simulink model "videomodel_V1"  (R2021a)
settings: Solver=VariableStepAuto  StartTime=0.0  StopTime=10.0  RelTol=1e-3
libraries: vexarmcortexlib x19, vexcommonlib x4
settings Model: Creator=Mihai Nicoara  LastModifiedBy=Mihai Nicoara

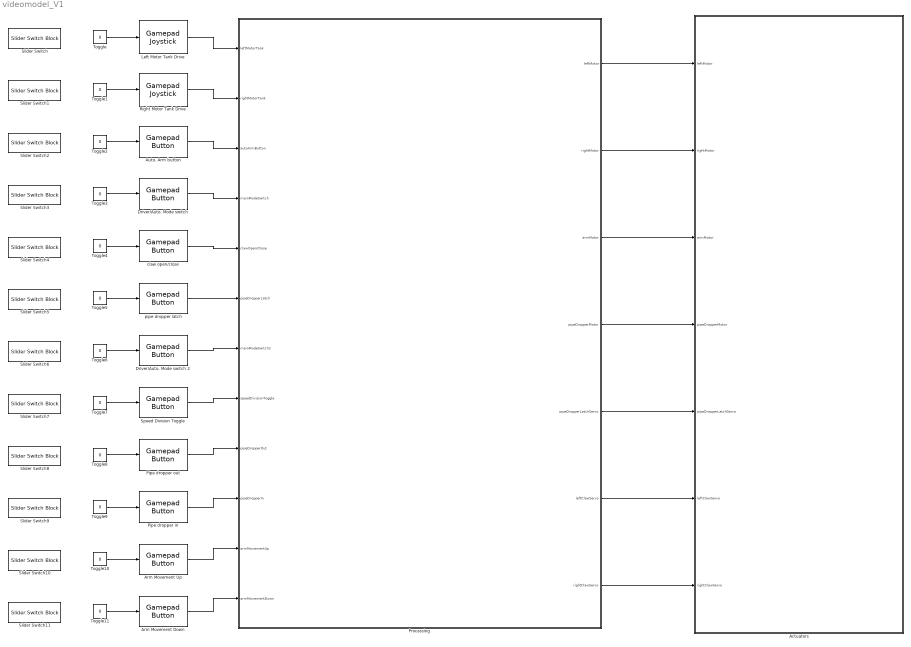
== system videomodel_V1 ==
  Actuators : Subsystem
  Arm Movement Down : vexarmcortexlib/Gamepad/Gamepad Button  joystick=1  chan=6  button56=Down  button78=Down  SimulationIn=on  SampleTime=0.02
      settings: SourceProductBaseCode=EC_VEX_MICRO
  Arm Movement Up : vexarmcortexlib/Gamepad/Gamepad Button  joystick=1  chan=6  button56=Up  button78=Down  SimulationIn=on  SampleTime=0.02
      settings: SourceProductBaseCode=EC_VEX_MICRO
  Auto. Arm button : vexarmcortexlib/Gamepad/Gamepad Button  joystick=1  chan=8  button56=Up  button78=Up  SimulationIn=on  SampleTime=0.02
      settings: SourceProductBaseCode=EC_VEX_MICRO
  Driver/Auto. Mode switch : vexarmcortexlib/Gamepad/Gamepad Button  joystick=1  chan=8  button56=Up  button78=Down  SimulationIn=on  SampleTime=0.02
      settings: SourceProductBaseCode=EC_VEX_MICRO
  Driver/Auto. Mode switch 2 : vexarmcortexlib/Gamepad/Gamepad Button  joystick=1  chan=7  button56=Up  button78=Down  SimulationIn=on  SampleTime=0.02
      settings: SourceProductBaseCode=EC_VEX_MICRO
  Left Motor Tank Drive : vexarmcortexlib/Gamepad/Gamepad Joystick  joystick=1  chan=3  SimulationIn=on  SampleTime=0.02
      settings: SourceProductBaseCode=EC_VEX_MICRO
  Pipe dropper in : vexarmcortexlib/Gamepad/Gamepad Button  joystick=1  chan=5  button56=Down  button78=Down  SimulationIn=on  SampleTime=0.02
      settings: SourceProductBaseCode=EC_VEX_MICRO
  Pipe dropper out : vexarmcortexlib/Gamepad/Gamepad Button  joystick=1  chan=5  button56=Up  button78=Down  SimulationIn=on  SampleTime=0.02
      settings: SourceProductBaseCode=EC_VEX_MICRO
  Processing : Subsystem
  Right Motor Tank Drive : vexarmcortexlib/Gamepad/Gamepad Joystick  joystick=1  chan=2  SimulationIn=on  SampleTime=0.02
      settings: SourceProductBaseCode=EC_VEX_MICRO
  Slider Switch{,1..11} (12 alike) : SliderSwitchBlock
      settings: Values={{'Off', 'On'}, [0 1]}
  Speed Division Toggle : vexarmcortexlib/Gamepad/Gamepad Button  joystick=1  chan=7  button56=Up  button78=Right  SimulationIn=on  SampleTime=0.02
      settings: SourceProductBaseCode=EC_VEX_MICRO
  Toggle{,1..11} (12 alike) : Constant  Value=0
      settings: OpenFcn=|
      | if strcmp('0',get_param(gcb, 'Value'))                        set_param(gcb, 'Value', '1');
      | else
      |             set_param(gcb, 'Value', '0');
      | end
  claw open/close : vexarmcortexlib/Gamepad/Gamepad Button  joystick=1  chan=8  button56=Up  button78=Right  SimulationIn=on  SampleTime=0.02
      settings: SourceProductBaseCode=EC_VEX_MICRO
  pipe dropper latch : vexarmcortexlib/Gamepad/Gamepad Button  joystick=1  chan=7  button56=Up  button78=Up  SimulationIn=on  SampleTime=0.02
      settings: SourceProductBaseCode=EC_VEX_MICRO
  wires:
  Toggle/1 -> Left Motor Tank Drive/1
  Toggle1/1 -> Right Motor Tank Drive/1
  Toggle3/1 -> Driver/Auto. Mode switch/1
  Toggle4/1 -> claw open/close/1
  Toggle5/1 -> pipe dropper latch/1
  Toggle6/1 -> Driver/Auto. Mode switch 2/1
  Toggle7/1 -> Speed Division Toggle/1
  Toggle8/1 -> Pipe dropper out/1
  Toggle9/1 -> Pipe dropper in/1
  Toggle10/1 -> Arm Movement Up/1
  Toggle11/1 -> Arm Movement Down/1
  Toggle2/1 -> Auto. Arm button/1
  Left Motor Tank Drive/1 -> Processing/1(leftMotorTank)
  Right Motor Tank Drive/1 -> Processing/2(rightMotorTank)
  Auto. Arm button/1 -> Processing/3(autoArmButton)
  Driver/Auto. Mode switch/1 -> Processing/4(mainModeSwitch)
  claw open/close/1 -> Processing/5(clawOpen/Close)
  pipe dropper latch/1 -> Processing/6(pipeDropperLatch)
  Driver/Auto. Mode switch 2/1 -> Processing/7(mainModeSwitch2)
  Speed Division Toggle/1 -> Processing/8(speedDivisionToggle)
  Pipe dropper out/1 -> Processing/9(pipeDropperOut)
  Pipe dropper in/1 -> Processing/10(pipeDropperIn)
  Arm Movement Up/1 -> Processing/11(armMovementUp)
  Arm Movement Down/1 -> Processing/12(armMovementDown)
  Processing/3(armMotor) -> Actuators/3(armMotor)
  Processing/4(pipeDropperMotor) -> Actuators/4(pipeDropperMotor)
  Processing/5(pipeDropperLatchServo) -> Actuators/5(pipeDropperLatchServo)
  Processing/6(leftClawServo) -> Actuators/6(leftClawServo)
  Processing/7(rightClawServo) -> Actuators/7(rightClawServo)
  Processing/2(rightMotor) -> Actuators/2(rightMotor)
  Processing/1(leftMotor) -> Actuators/1(leftMotor)

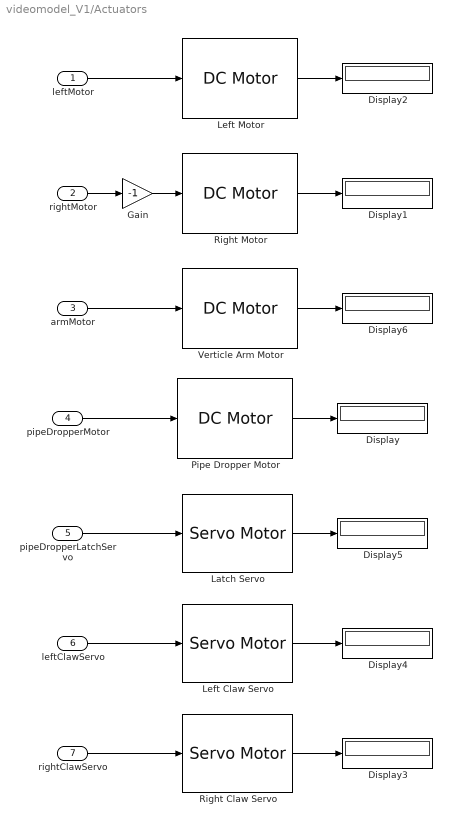
== system videomodel_V1/Actuators ==
  leftMotor : Inport
  rightMotor : Inport  Port=2
  armMotor : Inport  Port=3
  pipeDropperMotor : Inport  Port=4
  pipeDropperLatchServo : Inport  Port=5
  leftClawServo : Inport  Port=6
  rightClawServo : Inport  Port=7
  Display{,1..6} (7 alike) : Display
  Gain : Gain  Gain=-1
  Latch Servo : vexarmcortexlib/Actuators/Servo Motor  motor=8  scaleFactor=60/127  SimulationOut=on
      settings: SourceProductBaseCode=EC_VEX_MICRO
  Left Claw Servo : vexarmcortexlib/Actuators/Servo Motor  motor=5  scaleFactor=60/127  SimulationOut=on
      settings: SourceProductBaseCode=EC_VEX_MICRO
  Left Motor : vexarmcortexlib/Actuators/DC Motor  motor=9  scaleFactor=1/13.5  SimulationOut=on
      settings: SourceProductBaseCode=EC_VEX_MICRO
  Pipe Dropper Motor : vexarmcortexlib/Actuators/DC Motor  motor=4  scaleFactor=1/13.5  SimulationOut=on
      settings: SourceProductBaseCode=EC_VEX_MICRO
  Right Claw Servo : vexarmcortexlib/Actuators/Servo Motor  motor=3  scaleFactor=60/127  SimulationOut=on
      settings: SourceProductBaseCode=EC_VEX_MICRO
  Right Motor : vexarmcortexlib/Actuators/DC Motor  motor=2  scaleFactor=1/13.5  SimulationOut=on
      settings: SourceProductBaseCode=EC_VEX_MICRO
  Verticle Arm Motor : vexarmcortexlib/Actuators/DC Motor  motor=7  scaleFactor=1/13.5  SimulationOut=on
      settings: SourceProductBaseCode=EC_VEX_MICRO
  wires:
  Right Claw Servo/1 -> Display3/1
  pipeDropperMotor/1 -> Pipe Dropper Motor/1
  rightClawServo/1 -> Right Claw Servo/1
  Pipe Dropper Motor/1 -> Display/1
  Verticle Arm Motor/1 -> Display6/1
  Right Motor/1 -> Display1/1
  Latch Servo/1 -> Display5/1
  armMotor/1 -> Verticle Arm Motor/1
  pipeDropperLatchServo/1 -> Latch Servo/1
  rightMotor/1 -> Gain/1
  Gain/1 -> Right Motor/1
  Left Claw Servo/1 -> Display4/1
  leftClawServo/1 -> Left Claw Servo/1
  leftMotor/1 -> Left Motor/1
  Left Motor/1 -> Display2/1

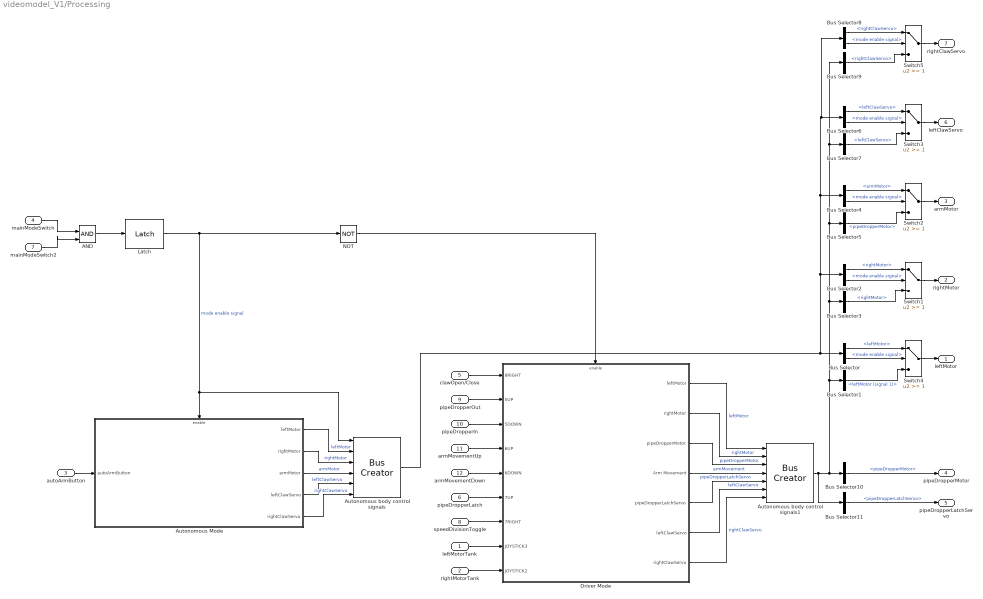
== system videomodel_V1/Processing ==
  leftMotorTank : Inport
  rightMotorTank : Inport  Port=2
  autoArmButton : Inport  Port=3
  mainModeSwitch : Inport  Port=4
  clawOpen/Close : Inport  Port=5
  pipeDropperLatch : Inport  Port=6
  mainModeSwitch2 : Inport  Port=7
  speedDivisionToggle : Inport  Port=8
  pipeDropperOut : Inport  Port=9
  pipeDropperIn : Inport  Port=10
  armMovementUp : Inport  Port=11
  armMovementDown : Inport  Port=12
  "AND " : Logic  IconShape=distinctive  AllPortsSameDT=off  OutDataTypeStr=boolean
  Autonomous Mode : Subsystem  TreatAsAtomicUnit=on
  Autonomous body control signals : BusCreator  Inputs=6
  Autonomous body control signals1 : BusCreator  Inputs=7
  Bus Selector : BusSelector  OutputSignals=leftMotor,mode enable signal
  Bus Selector1 : BusSelector  OutputSignals=leftMotor (signal 1)
  Bus Selector10 : BusSelector  OutputSignals=pipeDropperMotor
  Bus Selector11 : BusSelector  OutputSignals=pipeDropperLatchServo
  Bus Selector2 : BusSelector  OutputSignals=rightMotor,mode enable signal
  Bus Selector3 : BusSelector  OutputSignals=rightMotor
  Bus Selector4 : BusSelector  OutputSignals=armMotor,mode enable signal
  Bus Selector5 : BusSelector  OutputSignals=pipeDropperMotor
  Bus Selector6 : BusSelector  OutputSignals=leftClawServo,mode enable signal
  Bus Selector7 : BusSelector  OutputSignals=leftClawServo
  Bus Selector8 : BusSelector  OutputSignals=rightClawServo,mode enable signal
  Bus Selector9 : BusSelector  OutputSignals=rightClawServo
  Driver Mode : Subsystem  TreatAsAtomicUnit=on
  Latch : vexcommonlib/Latch  output0=off  BlockPlatform=vexarmcortex
      settings: SourceProductBaseCode=EC_VEX_MICRO,VEXV5
  NOT : Logic  Operator=NOT  IconShape=distinctive  AllPortsSameDT=off  OutDataTypeStr=boolean
  Switch{1..5} (5 alike) : Switch  Threshold=1
  leftMotor : Outport
  rightMotor : Outport  Port=2
  armMotor : Outport  Port=3
  pipeDropperMotor : Outport  Port=4
  pipeDropperLatchServo : Outport  Port=5
  leftClawServo : Outport  Port=6
  rightClawServo : Outport  Port=7
  wires:
  mainModeSwitch2/1 -> "AND "/2
  mainModeSwitch/1 -> "AND "/1
  "AND "/1 -> Latch/1
  Latch/1 -> NOT/1, Autonomous body control signals/1, Autonomous Mode/Enable  "mode enable signal"
  autoArmButton/1 -> Autonomous Mode/1(autoArmButton)
  NOT/1 -> Driver Mode/Enable
  clawOpen/Close/1 -> Driver Mode/1(8RIGHT)
  pipeDropperOut/1 -> Driver Mode/2(5UP)
  pipeDropperIn/1 -> Driver Mode/3(5DOWN)
  armMovementUp/1 -> Driver Mode/4(6UP)
  armMovementDown/1 -> Driver Mode/5(6DOWN)
  pipeDropperLatch/1 -> Driver Mode/6(7UP)
  speedDivisionToggle/1 -> Driver Mode/7(7RIGHT)
  leftMotorTank/1 -> Driver Mode/8(JOYSTICK3)
  rightMotorTank/1 -> Driver Mode/9(JOYSTICK2)
  Autonomous Mode/2(rightMotor) -> Autonomous body control signals/3  "rightMotor"
  Autonomous Mode/3(armMotor) -> Autonomous body control signals/4  "armMotor"
  Autonomous Mode/4(leftClawServo) -> Autonomous body control signals/5  "leftClawServo"
  Autonomous Mode/5(rightClawServo) -> Autonomous body control signals/6  "rightClawServo"
  Driver Mode/1(leftMotor) -> Autonomous body control signals1/1  "leftMotor"
  Driver Mode/2(rightMotor) -> Autonomous body control signals1/2  "rightMotor"
  Driver Mode/3(pipeDropperMotor) -> Autonomous body control signals1/3  "pipeDropperMotor"
  Driver Mode/5(pipeDropperLatchServo) -> Autonomous body control signals1/5  "pipeDropperLatchServo"
  Driver Mode/6(leftClawServo) -> Autonomous body control signals1/6  "leftClawServo"
  Driver Mode/7(rightClawServo) -> Autonomous body control signals1/7  "rightClawServo"
  Autonomous body control signals1/1 -> Bus Selector9/1, Bus Selector7/1, Bus Selector5/1, Bus Selector3/1, Bus Selector1/1, Bus Selector10/1, Bus Selector11/1
  Autonomous body control signals/1 -> Bus Selector8/1, Bus Selector6/1, Bus Selector4/1, Bus Selector2/1, Bus Selector/1
  Bus Selector1/1 -> Switch4/3  "<leftMotor (signal 1)>"
  Bus Selector/2 -> Switch4/2  "<mode enable signal>"
  Bus Selector/1 -> Switch4/1  "<leftMotor>"
  Switch4/1 -> leftMotor/1
  Driver Mode/4(Arm Movement) -> Autonomous body control signals1/4  "armMovement"
  Autonomous Mode/1(leftMotor) -> Autonomous body control signals/2  "leftMotor"
  Switch1/1 -> rightMotor/1
  Bus Selector2/1 -> Switch1/1  "<rightMotor>"
  Bus Selector2/2 -> Switch1/2  "<mode enable signal>"
  Bus Selector3/1 -> Switch1/3  "<rightMotor>"
  Bus Selector5/1 -> Switch2/3  "<pipeDropperMotor>"
  Bus Selector4/2 -> Switch2/2  "<mode enable signal>"
  Bus Selector4/1 -> Switch2/1  "<armMotor>"
  Switch2/1 -> armMotor/1
  Switch3/1 -> leftClawServo/1
  Bus Selector6/1 -> Switch3/1  "<leftClawServo>"
  Bus Selector6/2 -> Switch3/2  "<mode enable signal>"
  Bus Selector7/1 -> Switch3/3  "<leftClawServo>"
  Switch5/1 -> rightClawServo/1
  Bus Selector8/1 -> Switch5/1  "<rightClawServo>"
  Bus Selector8/2 -> Switch5/2  "<mode enable signal>"
  Bus Selector9/1 -> Switch5/3  "<rightClawServo>"
  Bus Selector10/1 -> pipeDropperMotor/1  "<pipeDropperMotor>"
  Bus Selector11/1 -> pipeDropperLatchServo/1  "<pipeDropperLatchServo>"

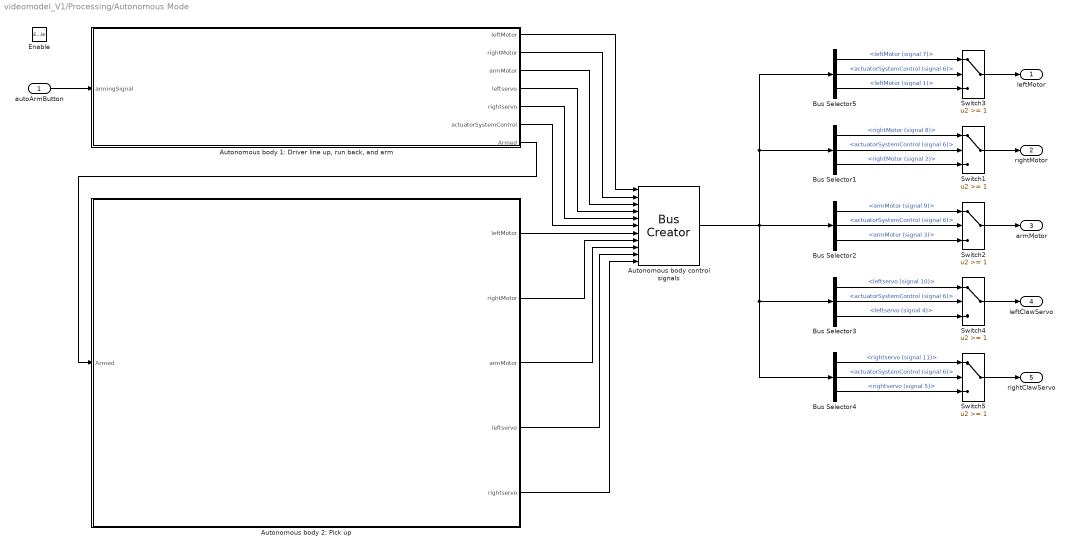
== system videomodel_V1/Processing/Autonomous Mode ==
  autoArmButton : Inport
  Enable : EnablePort  StatesWhenEnabling=reset
  "Autonomous body 1: Driver line up, run back, and arm" : Stateflow chart  TreatAsAtomicUnit=on
      settings: PortSchema="{\"entries\":[{\"content\":{\"sides\":[{\"content\":{\"connectorIds\":[\"In1\"]},\"type\":\"ConnectorPlacement.EquallySpacedRectSide\",\"uuid\":\"26c368e6-2070-416d-8296-f6cb4f90e07d\"},{\"content\":{\"connectorIds\":[\"Out7\",\"Out2\",\"Out1\",\"Out5\",\"Out4\",\"Out6\",\"Out3\"],\"side\":\"RIGHT\"},\"type\":\"ConnectorPlacement.EquallySpacedRectSide\",\"uuid\":\"e925f9e8-24eb-4129-a5ea-ee923b86028b\"},{\"content\":{\"connectorIds\":[],\"side\":\"TOP\"},\"type\":\"ConnectorPlacement.EquallySpacedRectSide\",\"uuid\":\"328c2cc5-1df2-40b9-96d3-d8939cd50370\"}]},\"type\":\"ConnectorPlacement.EquallySpacedConnector\",\"uuid\":\"f8afc3ae-2e44-461d-8e51-18dda479ef90\"}],\"packageUris\":[\"http://schema.mathworks.com/mf0/Connector/R2020b\"],\"version\":\"1.0\"}"
  Autonomous body 2: Pick up : Stateflow chart  TreatAsAtomicUnit=on
      settings: PortSchema="{\"entries\":[{\"content\":{\"sides\":[{\"content\":{\"connectorIds\":[\"In1\"]},\"type\":\"ConnectorPlacement.EquallySpacedRectSide\",\"uuid\":\"01bd6f1d-16cd-4d0a-aace-7294c8e32e1e\"},{\"content\":{\"connectorIds\":[\"Out1\",\"Out2\",\"Out3\",\"Out5\",\"Out4\"],\"side\":\"RIGHT\"},\"type\":\"ConnectorPlacement.EquallySpacedRectSide\",\"uuid\":\"acad459c-f867-4aff-8f10-4899709953d4\"},{\"content\":{\"connectorIds\":[],\"side\":\"TOP\"},\"type\":\"ConnectorPlacement.EquallySpacedRectSide\",\"uuid\":\"a3f1b2dd-e84f-4122-8883-ac3d505108ea\"}]},\"type\":\"ConnectorPlacement.EquallySpacedConnector\",\"uuid\":\"f33df9e5-376d-418a-b033-2b31451fa58c\"}],\"packageUris\":[\"http://schema.mathworks.com/mf0/Connector/R2020b\"],\"version\":\"1.0\"}"
  Autonomous body control signals : BusCreator  Inputs=11
  Bus Selector1 : BusSelector  OutputSignals=rightMotor (signal 8),actuatorSystemControl (signal 6),rightMotor (signal 2)
  Bus Selector2 : BusSelector  OutputSignals=armMotor (signal 9),actuatorSystemControl (signal 6),armMotor (signal 3)
  Bus Selector3 : BusSelector  OutputSignals=leftservo (signal 10),actuatorSystemControl (signal 6),leftservo (signal 4)
  Bus Selector4 : BusSelector  OutputSignals=rightservo (signal 11),actuatorSystemControl (signal 6),rightservo (signal 5)
  Bus Selector5 : BusSelector  OutputSignals=leftMotor (signal 7),actuatorSystemControl (signal 6),leftMotor (signal 1)
  Switch{1..5} (5 alike) : Switch  Threshold=1
  leftMotor : Outport
  rightMotor : Outport  Port=2
  armMotor : Outport  Port=3
  leftClawServo : Outport  Port=4
  rightClawServo : Outport  Port=5
  wires:
  autoArmButton/1 -> "Autonomous body 1: Driver line up, run back, and arm"/1(armingSignal)
  "Autonomous body 1: Driver line up, run back, and arm"/3(Armed) -> Autonomous body 2: Pick up/1(Armed)
  "Autonomous body 1: Driver line up, run back, and arm"/7(leftMotor) -> Autonomous body control signals/1
  "Autonomous body 1: Driver line up, run back, and arm"/2(rightMotor) -> Autonomous body control signals/2
  "Autonomous body 1: Driver line up, run back, and arm"/1(armMotor) -> Autonomous body control signals/3
  "Autonomous body 1: Driver line up, run back, and arm"/5(leftservo) -> Autonomous body control signals/4
  "Autonomous body 1: Driver line up, run back, and arm"/4(rightservo) -> Autonomous body control signals/5
  "Autonomous body 1: Driver line up, run back, and arm"/6(actuatorSystemControl) -> Autonomous body control signals/6
  Autonomous body 2: Pick up/1(leftMotor) -> Autonomous body control signals/7
  Autonomous body 2: Pick up/2(rightMotor) -> Autonomous body control signals/8
  Autonomous body 2: Pick up/3(armMotor) -> Autonomous body control signals/9
  Autonomous body 2: Pick up/5(leftservo) -> Autonomous body control signals/10
  Autonomous body 2: Pick up/4(rightservo) -> Autonomous body control signals/11
  Switch3/1 -> leftMotor/1
  Autonomous body control signals/1 -> Bus Selector1/1, Bus Selector5/1, Bus Selector4/1, Bus Selector3/1, Bus Selector2/1
  Bus Selector5/2 -> Switch3/2  "<actuatorSystemControl (signal 6)>"
  Bus Selector5/3 -> Switch3/3  "<leftMotor (signal 1)>"
  Bus Selector5/1 -> Switch3/1  "<leftMotor (signal 7)>"
  Bus Selector1/3 -> Switch1/3  "<rightMotor (signal 2)>"
  Bus Selector1/2 -> Switch1/2  "<actuatorSystemControl (signal 6)>"
  Bus Selector1/1 -> Switch1/1  "<rightMotor (signal 8)>"
  Switch1/1 -> rightMotor/1
  Switch2/1 -> armMotor/1
  Bus Selector2/1 -> Switch2/1  "<armMotor (signal 9)>"
  Bus Selector2/2 -> Switch2/2  "<actuatorSystemControl (signal 6)>"
  Bus Selector2/3 -> Switch2/3  "<armMotor (signal 3)>"
  Switch4/1 -> leftClawServo/1
  Bus Selector3/1 -> Switch4/1  "<leftservo (signal 10)>"
  Bus Selector3/2 -> Switch4/2  "<actuatorSystemControl (signal 6)>"
  Bus Selector3/3 -> Switch4/3  "<leftservo (signal 4)>"
  Switch5/1 -> rightClawServo/1
  Bus Selector4/1 -> Switch5/1  "<rightservo (signal 11)>"
  Bus Selector4/2 -> Switch5/2  "<actuatorSystemControl (signal 6)>"
  Bus Selector4/3 -> Switch5/3  "<rightservo (signal 5)>"

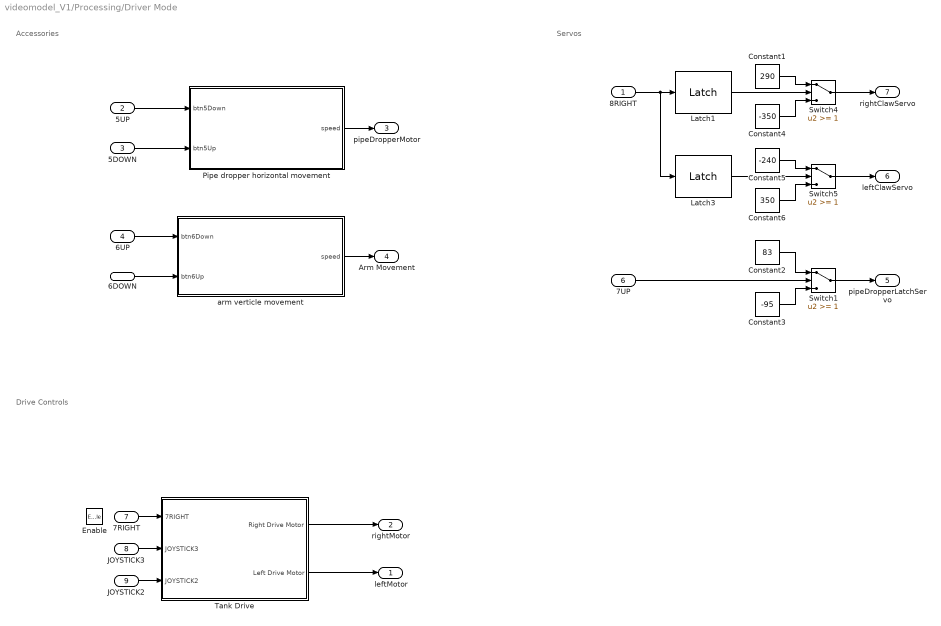
== system videomodel_V1/Processing/Driver Mode ==
  note: Accessories
  note: Drive Controls
  note: Servos
  8RIGHT : Inport
  5UP : Inport  Port=2
  5DOWN : Inport  Port=3
  6UP : Inport  Port=4
  6DOWN : Inport  Port=5
  7UP : Inport  Port=6
  7RIGHT : Inport  Port=7
  JOYSTICK3 : Inport  Port=8
  JOYSTICK2 : Inport  Port=9
  Enable : EnablePort
  Constant1 : Constant  Value=290
  Constant2 : Constant  Value=83
  Constant3 : Constant  Value=-95
  Constant4 : Constant  Value=-350
  Constant5 : Constant  Value=-240
  Constant6 : Constant  Value=350
  Latch1 : vexcommonlib/Latch  output0=off  BlockPlatform=vexarmcortex
      settings: SourceProductBaseCode=EC_VEX_MICRO,VEXV5
  Latch3 : vexcommonlib/Latch  output0=off  BlockPlatform=vexarmcortex
      settings: SourceProductBaseCode=EC_VEX_MICRO,VEXV5
  Pipe dropper horizontal movement : Stateflow chart  TreatAsAtomicUnit=on
  Switch1 : Switch  Threshold=1
  Switch4 : Switch  Threshold=1
  Switch5 : Switch  Threshold=1
  "Tank Drive " : Subsystem  TreatAsAtomicUnit=on
  arm verticle movement : Stateflow chart  TreatAsAtomicUnit=on
  leftMotor : Outport
  rightMotor : Outport  Port=2
  pipeDropperMotor : Outport  Port=3
  Arm Movement : Outport  Port=4
  pipeDropperLatchServo : Outport  Port=5
  leftClawServo : Outport  Port=6
  rightClawServo : Outport  Port=7
  wires:
  Constant6/1 -> Switch5/3
  Latch3/1 -> Switch5/2
  Constant5/1 -> Switch5/1
  Constant1/1 -> Switch4/1
  5UP/1 -> Pipe dropper horizontal movement/1(btn5Down)
  Switch4/1 -> rightClawServo/1
  5DOWN/1 -> Pipe dropper horizontal movement/2(btn5Up)
  8RIGHT/1 -> Latch3/1, Latch1/1
  7RIGHT/1 -> "Tank Drive "/1(7RIGHT)
  Constant3/1 -> Switch1/3
  Constant2/1 -> Switch1/1
  Switch5/1 -> leftClawServo/1
  7UP/1 -> Switch1/2
  JOYSTICK2/1 -> "Tank Drive "/3(JOYSTICK2)
  Latch1/1 -> Switch4/2
  JOYSTICK3/1 -> "Tank Drive "/2(JOYSTICK3)
  Switch1/1 -> pipeDropperLatchServo/1
  Pipe dropper horizontal movement/1(speed) -> pipeDropperMotor/1
  Constant4/1 -> Switch4/3
  6UP/1 -> arm verticle movement/1(btn6Down)
  6DOWN/1 -> arm verticle movement/2(btn6Up)
  "Tank Drive "/2(Left Drive Motor) -> leftMotor/1
  "Tank Drive "/1(Right Drive Motor) -> rightMotor/1
  arm verticle movement/1(speed) -> Arm Movement/1

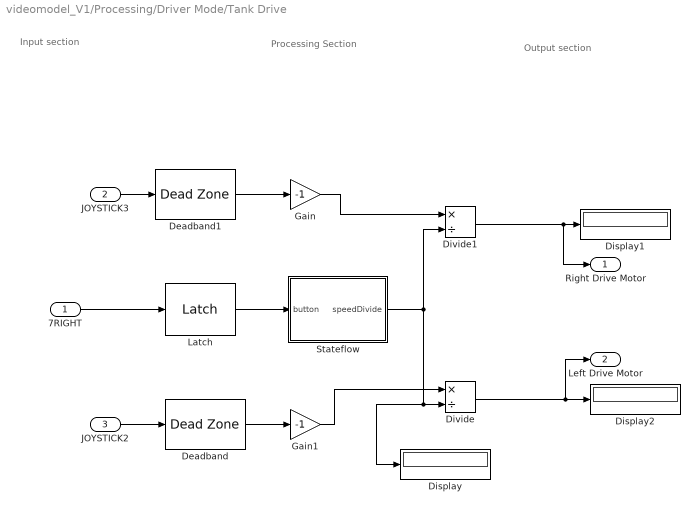
== system videomodel_V1/Processing/Driver Mode/Tank Drive  ==
  note: Output section
  note: Processing Section
  note: Input section
  7RIGHT : Inport
  JOYSTICK3 : Inport  Port=2
  JOYSTICK2 : Inport  Port=3
  Deadband : DeadZone  LowerValue=-9  UpperValue=9  SaturateOnIntegerOverflow=on
  Deadband1 : DeadZone  LowerValue=-9  UpperValue=9  SaturateOnIntegerOverflow=on
  Display : Display
  Display1 : Display
  Display2 : Display
  Divide : Product  Inputs=*/
  Divide1 : Product  Inputs=*/
  Gain : Gain  Gain=-1
  Gain1 : Gain  Gain=-1
  Latch : vexcommonlib/Latch  output0=off  BlockPlatform=vexarmcortex
      settings: SourceProductBaseCode=EC_VEX_MICRO,VEXV5
  Stateflow : Stateflow chart  TreatAsAtomicUnit=on
  Right Drive Motor : Outport
  Left Drive Motor : Outport  Port=2
  wires:
  7RIGHT/1 -> Latch/1
  Latch/1 -> Stateflow/1(button)
  Stateflow/1(speedDivide) -> Divide1/2, Display/1, Divide/2
  JOYSTICK3/1 -> Deadband1/1
  Divide1/1 -> Display1/1, Right Drive Motor/1
  Divide/1 -> Display2/1, Left Drive Motor/1
  JOYSTICK2/1 -> Deadband/1
  Gain/1 -> Divide1/1
  Gain1/1 -> Divide/1
  Deadband1/1 -> Gain/1
  Deadband/1 -> Gain1/1

== stateflow chart videomodel_V1/Processing/Driver Mode/arm verticle movement ==
  state ARMDOWN
    entry:
    speed = -50;
  state STOPPED
    entry:
    speed = 0;
  state ARMUP
    entry:
    speed = 100;
  (default) -> STOPPED
  STOPPED -> ARMUP [order 1] : [btn6Down == 0 && btn6Up == 1 ]
  STOPPED -> ARMDOWN [order 2] : [btn6Down == 1 && btn6Up == 0]
  ARMDOWN -> STOPPED [order 2] : [btn6Down == 0]
  ARMUP -> STOPPED [order 2] : [btn6Up == 0]
  ARMDOWN -> STOPPED [order 1] : [btn6Down == 1 && btn6Up == 1]
  ARMUP -> STOPPED [order 1] : [btn6Down == 1 && btn6Up == 1]
  data: speed output; btn6Down input; btn6Up input

== stateflow chart videomodel_V1/Processing/Autonomous Mode/Autonomous body 2: Pick up ==
  state Echo
    entry:
    leftMotor = 0;
    rightMotor = 0;
    armMotor = -60;
  state Armed
    entry:
    leftMotor = 0;
    rightMotor = 0;
    armMotor = 0;
  state Charlie
    entry:
    leftMotor = 0;
    rightMotor = 0;
    armMotor = 0;
  state Delta
    entry:
    leftMotor = -90;
    rightMotor = -90;
    armMotor = 0;
  state Foxtrot
    entry:
    leftMotor = 0;
    rightMotor = 0;
    armMotor =  0;
    rightservo = 200;
    leftservo = -200;
  state Golf
    entry:
    leftMotor = 0;
    rightMotor = 0;
    armMotor =  40;
    rightservo = 200;
    leftservo = -200;
  state Hotel
    entry:
    leftMotor = 115;
    rightMotor = 115;
    armMotor =  0;
    rightservo = 200;
    leftservo = -200;
  state India
    entry:
    leftMotor = 0;
    rightMotor = 0;
    armMotor =  0;
    rightservo = 200;
    leftservo = -200;
  (default) -> Armed
  Armed -> Charlie : [Armed == 1]
  Charlie -> Delta : [after(2.5,sec)]
  Delta -> Echo : [after(1.3,sec)]
  Echo -> Foxtrot : [after(1,sec)]
  Foxtrot -> Golf : [after(1,sec)]
  Golf -> Hotel : [after(0.8, sec)]
  Hotel -> India : [after(1.7,sec)]
  data: Armed input; leftMotor output; rightMotor output; armMotor output; rightservo output; leftservo output

== stateflow chart videomodel_V1/Processing/Autonomous Mode/Autonomous body 1: Driver line up, run back, and arm ==
  state Pre_Armed
    entry:
    leftMotor = 0;
    rightMotor = 0;
    armMotor = 0;
    Armed = 0;
    actuatorSystemControl = 0;
  state ARMED
    entry:
    Armed = 1;
    actuatorSystemControl = 0;
  state Alfa
    entry:
    leftMotor = 0;
    rightMotor = 0;
    armMotor = 50;
    rightservo = -350;
    leftservo = 350;
    Armed = 0;
  state Bravo
    entry:
    leftMotor = 130;
    rightMotor = 130;
    armMotor = 0;
    Armed = 0;
  state Start
    entry:
    leftMotor = 0;
    rightMotor = 0;
    armMotor = 0;
    rightservo = -350;
    leftservo = 350;
    Armed = 0;
  Pre_Armed -> ARMED : [armingSignal == 1]
  (default) -> Start
  Alfa -> Bravo : [after(1.3,sec)]
  Start -> Alfa : [after(2,sec)]
  Bravo -> Pre_Armed : [after(1.3,sec)]
  data: armMotor output; rightMotor output; armingSignal input; Armed output; rightservo output; leftservo output; actuatorSystemControl output; leftMotor output

== stateflow chart videomodel_V1/Processing/Driver Mode/Tank Drive /Stateflow ==
  state Full_Speed
    entry:
    speedDivide = 1
  state Slow_Speed
    entry:
    speedDivide = 2
  (default) -> Full_Speed
  Full_Speed -> Slow_Speed : [button]
  Slow_Speed -> Full_Speed : [button == 0]
  data: speedDivide output; button input

== stateflow chart videomodel_V1/Processing/Driver Mode/Pipe dropper horizontal movement ==
  state ARMDOWN
    entry:
    speed = -80;
  state STOPPED
    entry:
    speed = 0;
  state ARMUP
    entry:
    speed = 80;
  (default) -> STOPPED
  STOPPED -> ARMUP [order 1] : [btn5Down == 0 && btn5Up == 1 ]
  STOPPED -> ARMDOWN [order 2] : [btn5Down == 1 && btn5Up == 0]
  ARMDOWN -> STOPPED [order 2] : [btn5Down == 0]
  ARMUP -> STOPPED [order 2] : [btn5Up == 0]
  ARMDOWN -> STOPPED [order 1] : [btn5Down == 1 && btn5Up == 1]
  ARMUP -> STOPPED [order 1] : [btn5Down == 1 && btn5Up == 1]
  data: btn5Down input; btn5Up input; speed output
